simulink subsystem "EoMM"  (R2020a)
settings: Solver=VariableStepAuto  StartTime=0.0  StopTime=10.0  RelTol=1e-3
undefined symbols (not defined in the file): g, Ix, Ixz, Iy, Iz, m
settings Model: Creator=verti  LastModifiedBy=verti
settings DebuggingCC: SFMachineParentedDataDiag=error

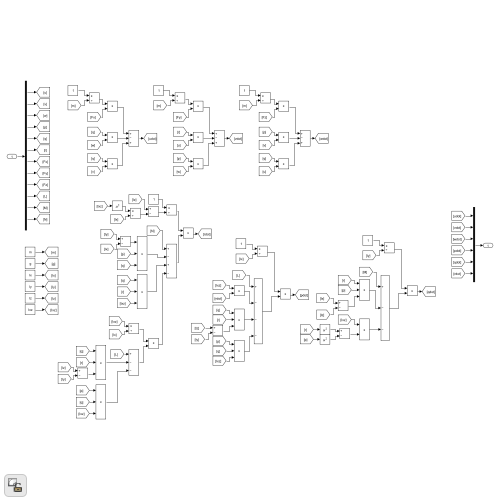
[thumbnail: Simulink's stored preview of the top-level diagram]
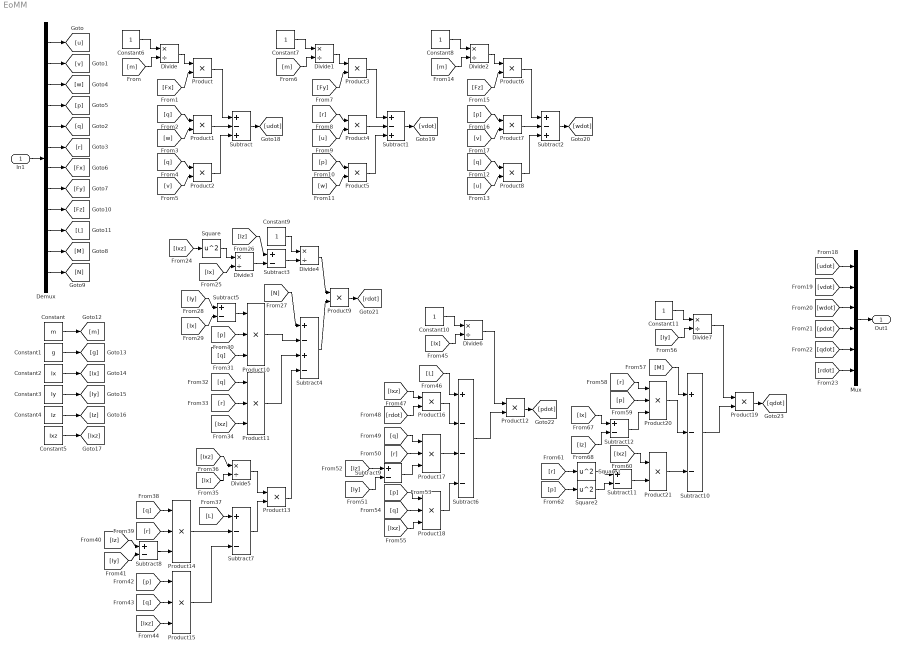
== system EoMM ==
  In1 : Inport  RequirementInfo={} %GIDa_42e59dd7_cc81_408d_b214_636d4c3dee52
  Constant : Constant  RequirementInfo={} %GIDa_98e7d0e0_a9ab_4f0b_9eff_a909e0454cff  Value=m
  Constant1 : Constant  RequirementInfo={} %GIDa_0eb29ca4_706a_459c_8611_c60782e4e9da  Value=g
  Constant10 : Constant  RequirementInfo={} %GIDa_2060170f_d90f_4e61_bda8_c9c99efe667d
  Constant11 : Constant  RequirementInfo={} %GIDa_5e565977_94e8_4ab0_8796_01e9a001e310
  Constant2 : Constant  RequirementInfo={} %GIDa_9652cfec_6219_4ca2_b6f7_a0c6f79b8a78  Value=Ix
  Constant3 : Constant  RequirementInfo={} %GIDa_122c7224_31bf_49e1_8298_d600f6830e4a  Value=Iy
  Constant4 : Constant  RequirementInfo={} %GIDa_202abd7c_95fa_4bb0_b41c_f13332bdf735  Value=Iz
  Constant5 : Constant  RequirementInfo={} %GIDa_ea437e0b_b64d_41bc_8aec_717ec757c633  Value=Ixz
  Constant6 : Constant  RequirementInfo={} %GIDa_59ff7bfa_b904_476c_87b1_57e3f41c69d4
  Constant7 : Constant  RequirementInfo={} %GIDa_8c7b753b_c63d_4693_9ffc_2b6a030754bb
  Constant8 : Constant  RequirementInfo={} %GIDa_da36ba7b_e82a_47d1_bf57_37cb584793f8
  Constant9 : Constant  RequirementInfo={} %GIDa_ab548ac4_c9d6_43ba_95f5_8e2711993162
  Demux : Demux  RequirementInfo={} %GIDa_c5049000_0a0f_4292_bbcc_1f3062cba7d6  Outputs=12
  Divide : Product  RequirementInfo={} %GIDa_0f72733c_eb82_4fc8_8f63_ec74304d15a4  Inputs=*/
  Divide1 : Product  RequirementInfo={} %GIDa_7076380a_0460_4d76_8b5c_ce13bdeb13f3  Inputs=*/
  Divide2 : Product  RequirementInfo={} %GIDa_d28d18c2_ce10_42a9_b133_d56ce9bdd16d  Inputs=*/
  Divide3 : Product  RequirementInfo={} %GIDa_bb3bd7f1_0b24_4e60_a653_e1e0159ddf9e  Inputs=*/
  Divide4 : Product  RequirementInfo={} %GIDa_2f285d2f_a61c_4c05_8c47_484a50ca08ae  Inputs=*/
  Divide5 : Product  RequirementInfo={} %GIDa_def20c2d_1a5f_4bc2_9f5d_75e15ef5b7de  Inputs=*/
  Divide6 : Product  RequirementInfo={} %GIDa_584581cc_1424_4b75_800c_077f2bbb2d2e  Inputs=*/
  Divide7 : Product  RequirementInfo={} %GIDa_d8dbe4d0_2425_427f_8a4d_d8dba8d069c6  Inputs=*/
  Mux : Mux  RequirementInfo={} %GIDa_b80b3029_3349_40ca_97d9_8b08c1515a1f  Inputs=6
  Product : Product  RequirementInfo={} %GIDa_88b83ead_2453_4de8_9544_71f38535c854
  Product1 : Product  RequirementInfo={} %GIDa_78be80e5_ad82_44dd_b95f_44864babe1ab
  Product10 : Product  RequirementInfo={} %GIDa_b6d4df9b_c0db_4a68_83d2_8dbd1b3741b2  Inputs=3
  Product11 : Product  RequirementInfo={} %GIDa_63ba5b4f_9e03_413a_be13_bc2e47f46a36  Inputs=3
  Product12 : Product  RequirementInfo={} %GIDa_a0f31848_a80a_4002_bf0f_03f0e8214674
  Product13 : Product  RequirementInfo={} %GIDa_0678e8cf_bd70_41c8_b79f_90919e641546
  Product14 : Product  RequirementInfo={} %GIDa_9210714b_a46f_4d2d_9c6a_9431b41e7013  Inputs=3
  Product15 : Product  RequirementInfo={} %GIDa_4da8b076_0f69_45ad_8b7e_11ff8ee07498  Inputs=3
  Product16 : Product  RequirementInfo={} %GIDa_7d1208c4_002a_4ef4_b2cf_609b6d3eaf04
  Product17 : Product  RequirementInfo={} %GIDa_10a15156_3552_4c20_a33d_d888651533d2  Inputs=3
  Product18 : Product  RequirementInfo={} %GIDa_0ab51921_9a7e_491a_a46d_0a4a8308d361  Inputs=3
  Product19 : Product  RequirementInfo={} %GIDa_dd722486_8643_4262_9188_087873e096a4
  Product2 : Product  RequirementInfo={} %GIDa_fe7c3ff1_d99a_4f34_ab6d_f01881b96355
  Product20 : Product  RequirementInfo={} %GIDa_ce1d4afa_50d2_4d53_b224_da8aa16c1694  Inputs=3
  Product21 : Product  RequirementInfo={} %GIDa_8b31bb0a_040d_45e8_8c2d_177830e1fcbf
  Product3 : Product  RequirementInfo={} %GIDa_45122bab_c2a0_4c64_9244_141b34772185
  Product4 : Product  RequirementInfo={} %GIDa_d039ed8a_cb91_4677_97dc_2b2992d7fe57
  Product5 : Product  RequirementInfo={} %GIDa_6ec128d3_f3fe_4c56_b873_8a4564d00f52
  Product6 : Product  RequirementInfo={} %GIDa_767ed524_9dfa_4f60_a202_256fc188a8a5
  Product7 : Product  RequirementInfo={} %GIDa_3811b28e_1d62_43b0_a495_8b3cd789e010
  Product8 : Product  RequirementInfo={} %GIDa_070a163c_5c8d_4fdb_ac7c_a44df70e0c90
  Product9 : Product  RequirementInfo={} %GIDa_482af599_38c1_43e8_a6ed_222bb26720be
  Square : Math  RequirementInfo={} %GIDa_9e105db7_f2bc_46bf_9d0b_b452bce3a4b9  Operator=square  SaturateOnIntegerOverflow=on
  Square1 : Math  RequirementInfo={} %GIDa_00617657_77b2_4079_8c46_84b1caf7cb38  Operator=square  SaturateOnIntegerOverflow=on
  Square2 : Math  RequirementInfo={} %GIDa_b6fd925a_1ea3_467c_ba1c_80727f419b20  Operator=square  SaturateOnIntegerOverflow=on
  Subtract : Sum  RequirementInfo={} %GIDa_baf0c23a_f2a9_4bae_b1f8_1b35b37ca232  Inputs=+-+
  Subtract1 : Sum  RequirementInfo={} %GIDa_979fe9f0_a731_43a3_ab77_e22a78b1d3b5  Inputs=+-+
  Subtract10 : Sum  RequirementInfo={} %GIDa_d177f9ce_cab1_4e93_b813_86de51844d93  Inputs=+--
  Subtract11 : Sum  RequirementInfo={} %GIDa_3958cfb7_b6bb_4297_92ce_865d109dbcdc  Inputs=+-
  Subtract12 : Sum  RequirementInfo={} %GIDa_654a3871_c3c0_456b_bba7_0741ad9d008c  Inputs=+-
  Subtract2 : Sum  RequirementInfo={} %GIDa_b4aa6628_361e_4bfc_b29f_19dd65e02a0e  Inputs=+-+
  Subtract3 : Sum  RequirementInfo={} %GIDa_b4b8707b_3492_4c57_9b91_c0402ec501f7  Inputs=+-
  Subtract4 : Sum  RequirementInfo={} %GIDa_90d09e63_f7da_4641_b29b_0b720594e21f  Inputs=+-+-
  Subtract5 : Sum  RequirementInfo={} %GIDa_53638e45_f791_4b94_b588_4eadac7ba981  Inputs=+-
  Subtract6 : Sum  RequirementInfo={} %GIDa_1f6ff7db_d90b_431f_a050_bcdb8de1a3fa  Inputs=+---
  Subtract7 : Sum  RequirementInfo={} %GIDa_c6ab96cf_3912_4073_852a_e580fe74e26b  Inputs=+--
  Subtract8 : Sum  RequirementInfo={} %GIDa_64a03a3e_258c_47b1_910f_6830289fee6b  Inputs=+-
  Subtract9 : Sum  RequirementInfo={} %GIDa_394e3019_c73d_458d_aee9_15a97890be83  Inputs=+-
  Out1 : Outport  RequirementInfo={} %GIDa_d14d5d32_aeee_47be_b0fb_4a0aa8e3f616
  wires:
  In1/1 -> Demux/1
  Demux/3 -> [w]
  Demux/1 -> [u]
  Demux/2 -> [v]
  Demux/4 -> [p]
  Demux/5 -> [q]
  Demux/6 -> [r]
  Demux/7 -> [Fx]
  Demux/12 -> [N]
  Demux/11 -> [M]
  Demux/10 -> [L]
  Demux/9 -> [Fz]
  Demux/8 -> [Fy]
  Constant/1 -> [m]
  Constant1/1 -> [g]
  Constant3/1 -> [Iy]
  Constant2/1 -> [Ix]
  Constant5/1 -> [Ixz]
  Constant4/1 -> [Iz]
  Constant6/1 -> Divide/1
  [m] -> Divide/2
  [Fx] -> Product/2
  Divide/1 -> Product/1
  [q] -> Product1/1
  [w] -> Product1/2
  [q] -> Product2/1
  [v] -> Product2/2
  Product2/1 -> Subtract/3
  Product/1 -> Subtract/1
  Product1/1 -> Subtract/2
  Subtract/1 -> [udot]
  Subtract1/1 -> [vdot]
  Product4/1 -> Subtract1/2
  Product3/1 -> Subtract1/1
  Product5/1 -> Subtract1/3
  [w] -> Product5/2
  [p] -> Product5/1
  [u] -> Product4/2
  [r] -> Product4/1
  Divide1/1 -> Product3/1
  [Fy] -> Product3/2
  [m] -> Divide1/2
  Constant7/1 -> Divide1/1
  Constant8/1 -> Divide2/1
  [m] -> Divide2/2
  [Fz] -> Product6/2
  Divide2/1 -> Product6/1
  [p] -> Product7/1
  [v] -> Product7/2
  [q] -> Product8/1
  [u] -> Product8/2
  Product8/1 -> Subtract2/3
  Product6/1 -> Subtract2/1
  Product7/1 -> Subtract2/2
  Subtract2/1 -> [wdot]
  [rdot] -> Mux/6
  Mux/1 -> Out1/1
  [udot] -> Mux/1
  [vdot] -> Mux/2
  [wdot] -> Mux/3
  [pdot] -> Mux/4
  [qdot] -> Mux/5
  [Ixz] -> Square/1
  Square/1 -> Divide3/1
  [Ix] -> Divide3/2
  [Iz] -> Subtract3/1
  Divide3/1 -> Subtract3/2
  Subtract3/1 -> Divide4/2
  Constant9/1 -> Divide4/1
  Divide4/1 -> Product9/1
  Subtract4/1 -> Product9/2
  [N] -> Subtract4/1
  [Iy] -> Subtract5/1
  [Ix] -> Subtract5/2
  Subtract5/1 -> Product10/1
  Product10/1 -> Subtract4/2
  [p] -> Product10/2
  [q] -> Product10/3
  [Ixz] -> Product11/3
  [r] -> Product11/2
  Product11/1 -> Subtract4/3
  [q] -> Product11/1
  [Ix] -> Divide5/2
  [Ixz] -> Divide5/1
  Product13/1 -> Subtract4/4
  Divide5/1 -> Product13/1
  Subtract7/1 -> Product13/2
  [L] -> Subtract7/1
  Product14/1 -> Subtract7/2
  Subtract8/1 -> Product14/3
  [q] -> Product14/1
  [r] -> Product14/2
  [Iz] -> Subtract8/1
  [Iy] -> Subtract8/2
  [q] -> Product15/2
  [p] -> Product15/1
  Product15/1 -> Subtract7/3
  [Ixz] -> Product15/3
  Product9/1 -> [rdot]
  Product12/1 -> [pdot]
  [Ix] -> Divide6/2
  Constant10/1 -> Divide6/1
  Divide6/1 -> Product12/1
  Subtract6/1 -> Product12/2
  [L] -> Subtract6/1
  [Ixz] -> Product16/1
  [rdot] -> Product16/2
  Product16/1 -> Subtract6/2
  Product17/1 -> Subtract6/3
  [q] -> Product17/1
  [r] -> Product17/2
  Subtract9/1 -> Product17/3
  [Iz] -> Subtract9/1
  [Iy] -> Subtract9/2
  [q] -> Product18/2
  [p] -> Product18/1
  [Ixz] -> Product18/3
  Product18/1 -> Subtract6/4
  [Ixz] -> Product21/1
  Product21/1 -> Subtract10/3
  Product20/1 -> Subtract10/2
  [M] -> Subtract10/1
  Subtract10/1 -> Product19/2
  Divide7/1 -> Product19/1
  Constant11/1 -> Divide7/1
  [Iy] -> Divide7/2
  Product19/1 -> [qdot]
  [r] -> Product20/1
  [p] -> Product20/2
  Subtract12/1 -> Product20/3
  [Ix] -> Subtract12/1
  [Iz] -> Subtract12/2
  Subtract11/1 -> Product21/2
  [r] -> Square1/1
  [p] -> Square2/1
  Square2/1 -> Subtract11/2
  Square1/1 -> Subtract11/1
